simulink library "ros2lib"  (R2025a)
settings: Solver=ode45  StartTime=0.0  StopTime=10.0  RelTol=1e-3  EnableMultiTasking=on
undefined symbols (not defined in the file): coder, count, data, data_SL_Info, datatype, encoding, encoding_SL_Info, fields, fields_SL_Info, header, height, name, name_SL_Info, offset, point_step, ros, row_step, width
libraries: $bdroot x3
(part 2 of 2)

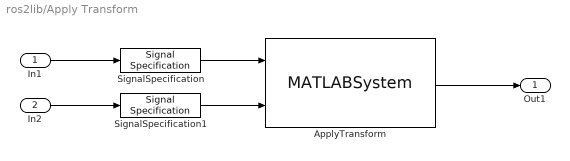
== system ros2lib/Apply Transform ==
  In1 : Inport
  In2 : Inport  Port=2
  ApplyTransform : MATLABSystem  System=ros.slros2.internal.block.ApplyTransform  EntityMsgType=geometry_msgs/QuaternionStamped  ModelName=ros2lib  BlockId=APTF_ros2lib_222  SLOutputBusName=SL_Bus_geometry_msgs_QuaternionStamped
      mask Type: ros.slros2.internal.block.ApplyTransform
  SignalSpecification : SignalSpecification  OutDataTypeStr=Bus: SL_Bus_geometry_msgs_TransformStamped  BusOutputAsStruct=on
      settings: LockScale=on
  SignalSpecification1 : SignalSpecification  OutDataTypeStr=Bus: SL_Bus_geometry_msgs_QuaternionStamped  BusOutputAsStruct=on
      settings: LockScale=on
  Out1 : Outport
  wires:
  In2/1 -> SignalSpecification1/1
  SignalSpecification1/1 -> ApplyTransform/2
  ApplyTransform/1 -> Out1/1
  In1/1 -> SignalSpecification/1
  SignalSpecification/1 -> ApplyTransform/1

== system ros2lib/Blank Message ==
  Constant : Constant  Value=0  OutDataTypeStr=Bus: SL_Bus_geometry_msgs_Point  SampleTime=SampleTime  LockScale=on
  Out : Outport  VectorParamsAs1DForOutWhenUnconnected=off  LockScale=on
  wires:
  Constant/1 -> Out/1

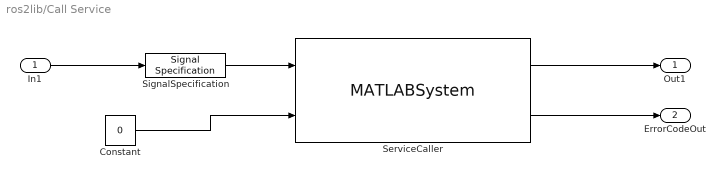
== system ros2lib/Call Service ==
  In1 : Inport
  Constant : Constant  Value=0  VectorParams1D=off  OutDataTypeStr=Bus: SL_Bus_std_srvs_EmptyResponse  SampleTime=-1
  ServiceCaller : MATLABSystem  System=ros.slros2.internal.block.ServiceCaller  QOSHistory=Keep last  QOSDepth=QOSDepth  QOSReliability=Reliable  QOSDurability=Volatile  QOSDeadline=QOSDeadline  QOSLifespan=QOSLifespan  QOSLiveliness=Automatic  QOSLeaseDuration=QOSLeaseDuration  ServiceName=/my_service  ServiceType=std_srvs/Empty  ConnectionTimeout=5  IsPersistentConnection=off  SLInputBusName=SL_Bus_std_srvs_EmptyRequest  SLOutputBusName=SL_Bus_std_srvs_EmptyResponse  ModelName=ros2lib  BlockId=ServCall_ros2lib_179
      mask Type: ros.slros2.internal.block.ServiceCaller
  SignalSpecification : SignalSpecification  OutDataTypeStr=Bus: SL_Bus_std_srvs_EmptyRequest  BusOutputAsStruct=on
      settings: LockScale=on
  Out1 : Outport
  ErrorCodeOut : Outport  Port=2
  wires:
  ServiceCaller/2 -> ErrorCodeOut/1
  Constant/1 -> ServiceCaller/2
  ServiceCaller/1 -> Out1/1
  In1/1 -> SignalSpecification/1
  SignalSpecification/1 -> ServiceCaller/1

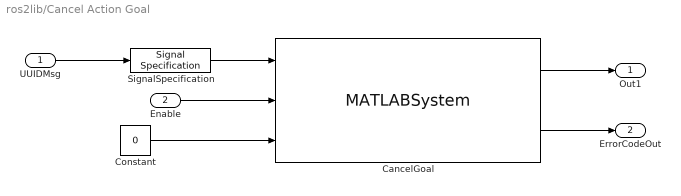
== system ros2lib/Cancel Action Goal ==
  UUIDMsg : Inport
  Enable : Inport  Port=2  OutDataTypeStr=boolean
  CancelGoal : MATLABSystem  System=ros.slros2.internal.block.CancelActionGoal  SLUUIDInputBusName=SL_Bus_unique_identifier_msgs_UUID  SLResponseOutputBusName=SL_Bus_action_msgs_CancelGoalResponse  ModelName=ros2lib  BlockId=ActCancel_ros2lib_244
      mask Type: ros.slros2.internal.block.CancelActionGoal
  Constant : Constant  Value=0  OutDataTypeStr=Bus: SL_Bus_action_msgs_CancelGoalResponse
  SignalSpecification : SignalSpecification  OutDataTypeStr=Bus: SL_Bus_unique_identifier_msgs_UUID  BusOutputAsStruct=on
      settings: LockScale=on
  Out1 : Outport
  ErrorCodeOut : Outport  Port=2
  wires:
  CancelGoal/2 -> ErrorCodeOut/1
  Constant/1 -> CancelGoal/3
  UUIDMsg/1 -> SignalSpecification/1
  Enable/1 -> CancelGoal/2
  SignalSpecification/1 -> CancelGoal/1
  CancelGoal/1 -> Out1/1

== system ros2lib/Get Transform ==
  Constant : Constant  Value=0  OutDataTypeStr=Bus: SL_Bus_geometry_msgs_TransformStamped  SampleTime=SampleTime
  SourceBlock : MATLABSystem  System=ros.slros2.internal.block.GetTransform  SLBusName=SL_Bus_geometry_msgs_TransformStamped  DynamicQoSHistory=Keep last  DynamicQoSDepth=DynamicQoSDepth  DynamicQoSReliability=Reliable  DynamicQoSDurability=Volatile  DynamicQOSDeadline=DynamicQoSDeadline  DynamicQOSLifespan=DynamicQoSLifespan  DynamicQOSLiveliness=Automatic  DynamicQOSLeaseDuration=DynamicQoSLeaseDuration  StaticQoSHistory=Keep last  StaticQoSDepth=StaticQoSDepth  StaticQoSReliability=Reliable  StaticQoSDurability=Volatile  StaticQOSDeadline=StaticQoSDeadline  StaticQOSLifespan=StaticQoSLifespan  StaticQOSLiveliness=Automatic  StaticQOSLeaseDuration=StaticQoSLeaseDuration  OutputFormat=bus  SampleTime=-1  ModelName=ros2lib  BlockId=TF_ros2lib_223
      mask Type: ros.slros2.internal.block.GetTransform
  Out1 : Outport
  Out2 : Outport  Port=2
  wires:
  Constant/1 -> SourceBlock/1
  SourceBlock/1 -> Out1/1
  SourceBlock/2 -> Out2/1

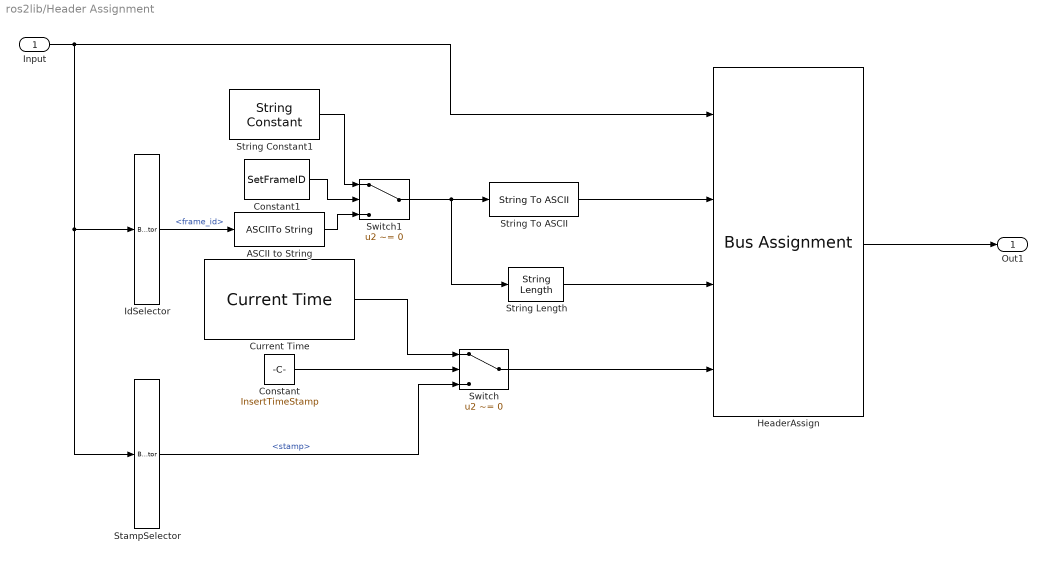
== system ros2lib/Header Assignment ==
  Input : Inport
  ASCII to String : ASCIIToString
  Constant : Constant  Value=InsertTimeStamp
  Constant1 : Constant  Value=SetFrameID
  Current Time : $bdroot/Current Time  OutputFormat=bus  SampleTime=-1  ModelName=tt
  HeaderAssign : BusAssignment  AssignedSignals=header.frame_id,header.frame_id_SL_Info.CurrentLength,header.stamp
  IdSelector : BusSelector  OutputSignals=header.frame_id
  StampSelector : BusSelector  OutputSignals=header.stamp
  String Constant1 : StringConstant  String=FrameID
  String Length : StringLength
  String To ASCII : StringToASCII  OutputVectorSize=128
  Switch : Switch  Criteria=u2 ~= 0  Threshold=1.5  SaturateOnIntegerOverflow=off  InputSameDT=off
  Switch1 : Switch  Criteria=u2 ~= 0  Threshold=1.5  SaturateOnIntegerOverflow=off  InputSameDT=off
  Out1 : Outport
  wires:
  Switch/1 -> HeaderAssign/4
  StampSelector/1 -> Switch/3  "<stamp>"
  Constant1/1 -> Switch1/2
  Constant/1 -> Switch/2
  String Length/1 -> HeaderAssign/3
  String Constant1/1 -> Switch1/1
  Switch1/1 -> String Length/1, String To ASCII/1
  Current Time/1 -> Switch/1
  String To ASCII/1 -> HeaderAssign/2
  ASCII to String/1 -> Switch1/3
  IdSelector/1 -> ASCII to String/1  "<frame_id>"
  HeaderAssign/1 -> Out1/1
  Input/1 -> StampSelector/1, IdSelector/1, HeaderAssign/1

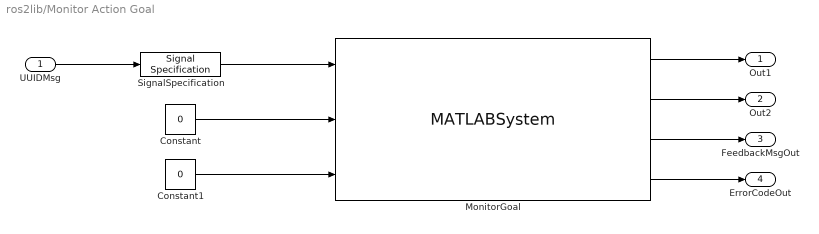
== system ros2lib/Monitor Action Goal ==
  UUIDMsg : Inport
  Constant : Constant  Value=0  OutDataTypeStr=Bus: SL_Bus_example_interfaces_FibonacciResult
  Constant1 : Constant  Value=0  OutDataTypeStr=Bus: SL_Bus_example_interfaces_FibonacciFeedback
  MonitorGoal : MATLABSystem  System=ros.slros2.internal.block.MonitorActionGoal  ActionName=/fibonacci  ActionType=example_interfaces/Fibonacci  SLUUIDInputBusName=SL_Bus_unique_identifier_msgs_UUID  SLFeedbackOutputBusName=SL_Bus_example_interfaces_FibonacciFeedback  SLResultOutputBusName=SL_Bus_example_interfaces_FibonacciResult  ModelName=ros2lib  BlockId=ActSend_ros2lib_226
      mask Type: ros.slros2.internal.block.MonitorActionGoal
  SignalSpecification : SignalSpecification  OutDataTypeStr=Bus: SL_Bus_unique_identifier_msgs_UUID  BusOutputAsStruct=on
      settings: LockScale=on
  Out1 : Outport
  Out2 : Outport  Port=2
  FeedbackMsgOut : Outport  Port=3
  ErrorCodeOut : Outport  Port=4
  wires:
  UUIDMsg/1 -> SignalSpecification/1
  Constant/1 -> MonitorGoal/2
  MonitorGoal/1 -> Out1/1
  MonitorGoal/2 -> Out2/1
  SignalSpecification/1 -> MonitorGoal/1
  MonitorGoal/3 -> FeedbackMsgOut/1
  Constant1/1 -> MonitorGoal/3
  MonitorGoal/4 -> ErrorCodeOut/1

== system ros2lib/Publish ==
  In1 : Inport  LockScale=on
  SignalSpecification : SignalSpecification  OutDataTypeStr=Bus: SL_Bus_geometry_msgs_Point  BusOutputAsStruct=on
      settings: LockScale=on
  SinkBlock : MATLABSystem  System=ros.slros2.internal.block.Publisher  QOSHistory=Keep last  QOSDepth=QOSDepth  QOSReliability=Reliable  QOSDurability=Volatile  QOSDeadline=QOSDeadline  QOSLifespan=QOSLifespan  QOSLiveliness=Automatic  QOSLeaseDuration=QOSLeaseDuration  ROSTopic=/my_topic  ROSMessageType=geometry_msgs/Point  SLBusName=SL_Bus_geometry_msgs_Point  ModelName=ros2lib  BlockId=Pub_ros2lib_156
      mask Type: ros.slros2.internal.block.Publisher
  wires:
  SignalSpecification/1 -> SinkBlock/1
  In1/1 -> SignalSpecification/1

== system ros2lib/Read Data ==
  SourceBlock : MATLABSystem  System=ros.slros2.internal.block.ReadData  LogfileType=rosbag2  Topic=/my_topic  SampleTime=sampleTime  ModelName=ros2lib
      mask Type: ros.slros2.internal.block.ReadData
  Out1 : Outport
  Out2 : Outport  Port=2
  wires:
  SourceBlock/2 -> Out2/1
  SourceBlock/1 -> Out1/1

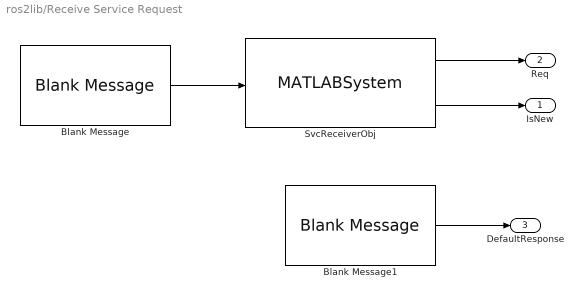
== system ros2lib/Receive Service Request ==
  Blank Message : $bdroot/Blank Message  messageClass=Service Request  entityType=std_srvs/Empty  messageType=std_srvs/EmptyRequest  SampleTime=SampleTime
  Blank Message1 : $bdroot/Blank Message  messageClass=Service Response  entityType=std_srvs/Empty  messageType=std_srvs/EmptyResponse  SampleTime=SampleTime
  SvcReceiverObj : MATLABSystem  System=ros.slros2.internal.block.SvcRequestReceiver  SLBusName=SL_Bus_std_srvs_EmptyRequest  ModelName=ros2lib  ServiceName=/my_service  ServiceType=std_srvs/Empty  BlockId=ServRec_ros2lib_224  QOSHistory=Keep last  QOSDepth=QOSDepth  QOSReliability=Reliable  QOSDurability=Volatile  QOSDeadline=QOSDeadline  QOSLifespan=QOSLifespan  QOSLiveliness=Automatic  QOSLeaseDuration=QOSLeaseDuration
      mask Type: ros.slros2.internal.block.SvcRequestReceiver
  IsNew : Outport
  Req : Outport  Port=2
  DefaultResponse : Outport  Port=3
  wires:
  Blank Message1/1 -> DefaultResponse/1
  Blank Message/1 -> SvcReceiverObj/1
  SvcReceiverObj/1 -> Req/1
  SvcReceiverObj/2 -> IsNew/1

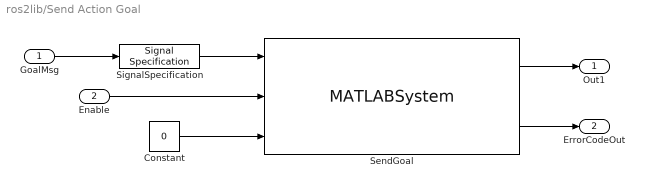
== system ros2lib/Send Action Goal ==
  GoalMsg : Inport
  Enable : Inport  Port=2  OutDataTypeStr=boolean
  Constant : Constant  Value=0  OutDataTypeStr=Bus: SL_Bus_unique_identifier_msgs_UUID
  SendGoal : MATLABSystem  System=ros.slros2.internal.block.SendActionGoal  ActionType=example_interfaces/Fibonacci  OutputROSMessageType=unique_identifier_msgs/UUID  SLUUIDOutputBusName=SL_Bus_unique_identifier_msgs_UUID  GoalServiceQoSHistory=Keep last  GoalServiceQoSDepth=GoalServiceQoSDepth  GoalServiceQoSReliability=Reliable  GoalServiceQoSDurability=Volatile  GoalServiceQoSDeadline=GoalServiceQoSDeadline  GoalServiceQoSLifespan=GoalServiceQoSLifespan  GoalServiceQoSLiveliness=Automatic  GoalServiceQoSLeaseDuration=GoalServiceQoSLeaseDuration  ResultServiceQoSHistory=Keep last  ResultServiceQoSDepth=ResultServiceQoSDepth  ResultServiceQoSReliability=Reliable  ResultServiceQoSDurability=Volatile  ResultServiceQoSDeadline=ResultServiceQoSDeadline  ResultServiceQoSLifespan=ResultServiceQoSLifespan  ResultServiceQoSLiveliness=Automatic  ResultServiceQoSLeaseDuration=ResultServiceQoSLeaseDuration  CancelServiceQoSHistory=Keep last  CancelServiceQoSDepth=CancelServiceQoSDepth  CancelServiceQoSReliability=Reliable  CancelServiceQoSDurability=Volatile  CancelServiceQoSDeadline=CancelServiceQoSDeadline  CancelServiceQoSLifespan=CancelServiceQoSLifespan  CancelServiceQoSLiveliness=Automatic  CancelServiceQoSLeaseDuration=CancelServiceQoSLeaseDuration  FeedbackTopicQoSHistory=Keep last  FeedbackTopicQoSDepth=FeedbackTopicQoSDepth  FeedbackTopicQoSReliability=Reliable  FeedbackTopicQoSDurability=Volatile  FeedbackTopicQoSDeadline=FeedbackTopicQoSDeadline  FeedbackTopicQoSLifespan=FeedbackTopicQoSLifespan  FeedbackTopicQoSLiveliness=Automatic  FeedbackTopicQoSLeaseDuration=FeedbackTopicQoSLeaseDuration  StatusTopicQoSHistory=Keep last  StatusTopicQoSDepth=StatusTopicQoSDepth  StatusTopicQoSReliability=Reliable  StatusTopicQoSDurability=Transient local  StatusTopicQoSDeadline=StatusTopicQoSDeadline  StatusTopicQoSLifespan=StatusTopicQoSLifespan  StatusTopicQoSLiveliness=Automatic  StatusTopicQoSLeaseDuration=StatusTopicQoSLeaseDuration  ActionName=/fibonacci  SLGoalInputBusName=SL_Bus_example_interfaces_FibonacciGoal  ModelName=ros2lib  BlockId=ActSend_ros2lib_226
      mask Type: ros.slros2.internal.block.SendActionGoal
  SignalSpecification : SignalSpecification  OutDataTypeStr=Bus: SL_Bus_example_interfaces_FibonacciGoal  BusOutputAsStruct=on
      settings: LockScale=on
  Out1 : Outport
  ErrorCodeOut : Outport  Port=2
  wires:
  SendGoal/1 -> Out1/1
  Constant/1 -> SendGoal/3
  SignalSpecification/1 -> SendGoal/1
  Enable/1 -> SendGoal/2
  GoalMsg/1 -> SignalSpecification/1
  SendGoal/2 -> ErrorCodeOut/1

== system ros2lib/Send Service Response ==
  resp : Inport
  SignalSpecification : SignalSpecification  OutDataTypeStr=Bus: SL_Bus_std_srvs_EmptyResponse  BusOutputAsStruct=on
      settings: LockScale=on
  SvcSenderObj : MATLABSystem  System=ros.slros2.internal.block.SvcResponseSender  ModelName=ros2lib  ServiceName=/my_service  ServiceType=std_srvs/Empty  BlockId=ServRec_ros2lib_224
      mask Type: ros.slros2.internal.block.SvcResponseSender
  wires:
  SignalSpecification/1 -> SvcSenderObj/1
  resp/1 -> SignalSpecification/1

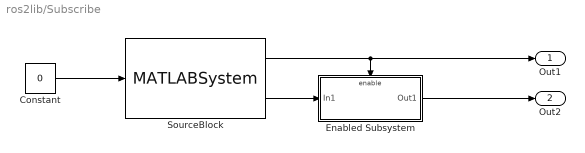
== system ros2lib/Subscribe ==
  Constant : Constant  Value=0  OutDataTypeStr=Bus: SL_Bus_geometry_msgs_Point  SampleTime=sampleTime  LockScale=on
  Enabled Subsystem : Subsystem  TreatAsAtomicUnit=on
  SourceBlock : MATLABSystem  System=ros.slros2.internal.block.Subscriber  QOSHistory=Keep last  QOSDepth=QOSDepth  QOSReliability=Reliable  QOSDurability=Volatile  QOSDeadline=QOSDeadline  QOSLifespan=QOSLifespan  QOSLiveliness=Automatic  QOSLeaseDuration=QOSLeaseDuration  ROSTopic=/my_topic  ROSMessageType=geometry_msgs/Point  SLBusName=SL_Bus_geometry_msgs_Point  ModelName=ros2lib  BlockId=Sub_ros2lib_139
      mask Type: ros.slros2.internal.block.Subscriber
  Out1 : Outport  VectorParamsAs1DForOutWhenUnconnected=off
  Out2 : Outport  Port=2  VectorParamsAs1DForOutWhenUnconnected=off
  wires:
  SourceBlock/1 -> Enabled Subsystem/Enable, Out1/1
  SourceBlock/2 -> Enabled Subsystem/1(In1)
  Constant/1 -> SourceBlock/1
  Enabled Subsystem/1(Out1) -> Out2/1

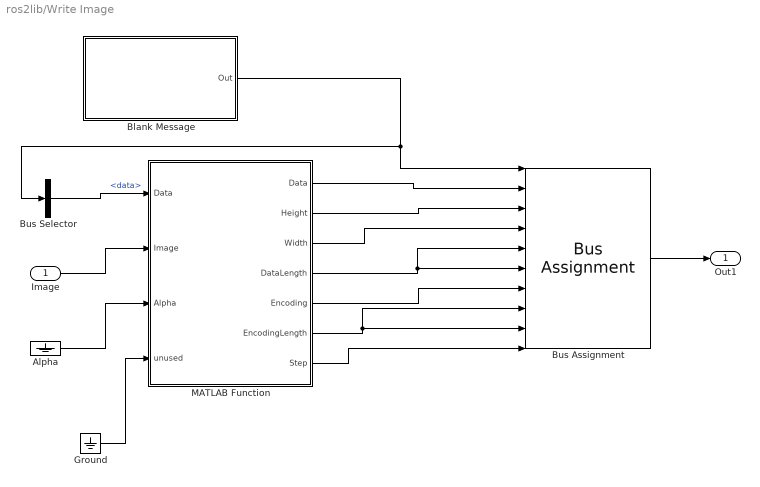
== system ros2lib/Write Image ==
  Image : Inport
  Alpha : Ground
  Blank Message : Subsystem  LoadFcn=ros.slros2.internal.block.MessageBlockMask.messageLoadFcn(gcb);  InitFcn=ros.slros.internal.block.errorIfBlocksConflict(bdroot(gcb));  mask(ROS2 Blank Message){messageClass=Message, entityType=sensor_msgs/Image, messageType=sensor_msgs/Image, SampleTime=inf}
      mask prompts: messageClass "ros:slros:blockmask:MessageClassPrompt"; entityType "ros:slros:blockmask:TypePrompt"; messageType "ros:slros:blockmask:FullTypePrompt"; SampleTime "Simulink:blkprm_prompts:AllSrcBlksSampleTime"
      mask help: ros:slros2:blockmask:BlankMsgDescription
      mask init:
      | ros.slros2.internal.block.MessageBlockMask.dispatch('maskInitialize', gcb);
      settings: ModelCloseFcn=ros.slros2.internal.bus.Util.clearSLBusesInGlobalScope();
      mask Help: eval('ros.slros.internal.helpview(''ros2BlankMsgBlock'')');
      mask TypeOptions messageClass: ros:slros:blockmask:MessageType_Msg | ros:slros:blockmask:MessageType_SrvReq | ros:slros:blockmask:MessageType_SrvResp
      mask Callback messageClass: ros.slros2.internal.block.MessageBlockMask.dispatch('messageClassChange', gcb);
      mask Callback entityType: ros.slros2.internal.block.MessageBlockMask.dispatch('entityTypeEdit', gcb);
      mask TypeOptions SampleTime: Constant/SampleTime
      mask DialogControl messageClass Prompt: Class:
      mask DialogControl entityType Prompt: Type:
      mask DialogControl id_msgTypeSelectBtn Prompt: ros:slros:blockmask:SelectPrompt
      mask DialogControl id_msgTypeSelectBtn Callback: ros.slros2.internal.block.MessageBlockMask.dispatch('selectButtonPressed', gcb);
      mask DialogControl messageType Prompt: Fully resolved type:
      mask DialogControl SampleTime Prompt: Sample time:
      mask Display: color('black');
  Bus Assignment : BusAssignment  AssignedSignals=data,height,width,data_SL_Info.CurrentLength,data_SL_Info.ReceivedLength,encoding,encoding_SL_Info.CurrentLength,encoding_SL_Info.ReceivedLength,step
  Bus Selector : BusSelector  OutputSignals=data
  Ground : Ground
  MATLAB Function : MATLAB Function  TreatAsAtomicUnit=on
  Out1 : Outport
  wires:
  MATLAB Function/1(Data) -> Bus Assignment/2
  MATLAB Function/3(Width) -> Bus Assignment/4
  MATLAB Function/5(Encoding) -> Bus Assignment/7
  Blank Message/1(Out) -> Bus Selector/1, Bus Assignment/1
  Bus Assignment/1 -> Out1/1
  MATLAB Function/2(Height) -> Bus Assignment/3
  Bus Selector/1 -> MATLAB Function/1("Data ")  "<data>"
  MATLAB Function/7(Step) -> Bus Assignment/10
  MATLAB Function/6(EncodingLength) -> Bus Assignment/8, Bus Assignment/9
  MATLAB Function/4(DataLength) -> Bus Assignment/5, Bus Assignment/6
  Image/1 -> MATLAB Function/2(Image)
  Alpha/1 -> MATLAB Function/3(Alpha)
  Ground/1 -> MATLAB Function/4(unused)

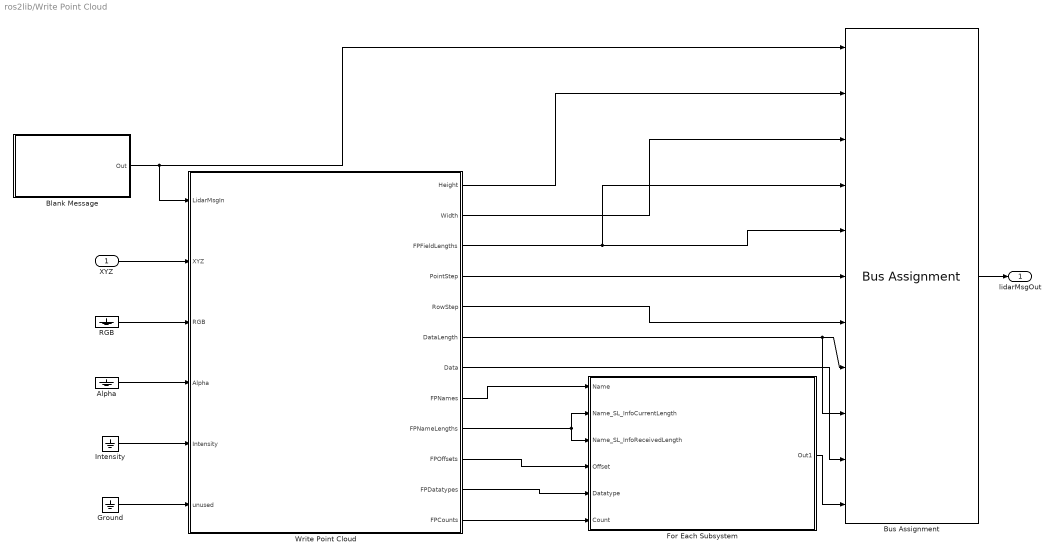
== system ros2lib/Write Point Cloud ==
  XYZ : Inport
  Alpha : Ground
  Blank Message : Subsystem  LoadFcn=ros.slros2.internal.block.MessageBlockMask.messageLoadFcn(gcb);  InitFcn=ros.slros.internal.block.errorIfBlocksConflict(bdroot(gcb));  mask(ROS2 Blank Message){messageClass=Message, entityType=sensor_msgs/PointCloud2, messageType=sensor_msgs/PointCloud2, SampleTime=inf}
      mask prompts: messageClass "ros:slros:blockmask:MessageClassPrompt"; entityType "ros:slros:blockmask:TypePrompt"; messageType "ros:slros:blockmask:FullTypePrompt"; SampleTime "Simulink:blkprm_prompts:AllSrcBlksSampleTime"
      mask help: ros:slros2:blockmask:BlankMsgDescription
      mask init:
      | ros.slros2.internal.block.MessageBlockMask.dispatch('maskInitialize', gcb);
      settings: ModelCloseFcn=ros.slros2.internal.bus.Util.clearSLBusesInGlobalScope();
      mask Help: eval('ros.slros.internal.helpview(''ros2BlankMsgBlock'')');
      mask TypeOptions messageClass: ros:slros:blockmask:MessageType_Msg | ros:slros:blockmask:MessageType_SrvReq | ros:slros:blockmask:MessageType_SrvResp
      mask Callback messageClass: ros.slros2.internal.block.MessageBlockMask.dispatch('messageClassChange', gcb);
      mask Callback entityType: ros.slros2.internal.block.MessageBlockMask.dispatch('entityTypeEdit', gcb);
      mask TypeOptions SampleTime: Constant/SampleTime
      mask DialogControl messageClass Prompt: Class:
      mask DialogControl entityType Prompt: Type:
      mask DialogControl id_msgTypeSelectBtn Prompt: ros:slros:blockmask:SelectPrompt
      mask DialogControl id_msgTypeSelectBtn Callback: ros.slros2.internal.block.MessageBlockMask.dispatch('selectButtonPressed', gcb);
      mask DialogControl messageType Prompt: Fully resolved type:
      mask DialogControl SampleTime Prompt: Sample time:
      mask Display: color('black');
  Bus Assignment : BusAssignment  AssignedSignals=height,width,fields_SL_Info.CurrentLength,fields_SL_Info.ReceivedLength,point_step,row_step,data_SL_Info.CurrentLength,data_SL_Info.ReceivedLength,data,fields
  For Each Subsystem : Subsystem  TreatAsAtomicUnit=on
  Ground : Ground
  Intensity : Ground
  RGB : Ground
  Write Point Cloud : MATLAB Function  TreatAsAtomicUnit=on
  lidarMsgOut : Outport
  wires:
  Bus Assignment/1 -> lidarMsgOut/1
  Write Point Cloud/12(FPCounts) -> For Each Subsystem/6(Count)
  Write Point Cloud/11(FPDatatypes) -> For Each Subsystem/5(Datatype)
  Write Point Cloud/10(FPOffsets) -> For Each Subsystem/4(Offset)
  Write Point Cloud/9(FPNameLengths) -> For Each Subsystem/2(Name_SL_InfoCurrentLength), For Each Subsystem/3(Name_SL_InfoReceivedLength)
  Write Point Cloud/8(FPNames) -> For Each Subsystem/1(Name)
  Write Point Cloud/7(Data) -> Bus Assignment/10
  For Each Subsystem/1(Out1) -> Bus Assignment/11
  Write Point Cloud/6(DataLength) -> Bus Assignment/8, Bus Assignment/9
  Write Point Cloud/5(RowStep) -> Bus Assignment/7
  Write Point Cloud/3(FPFieldLengths) -> Bus Assignment/5, Bus Assignment/4
  Intensity/1 -> Write Point Cloud/5(Intensity)
  Alpha/1 -> Write Point Cloud/4(Alpha)
  Ground/1 -> Write Point Cloud/6(unused)
  Write Point Cloud/2(Width) -> Bus Assignment/3
  RGB/1 -> Write Point Cloud/3(RGB)
  Write Point Cloud/1(Height) -> Bus Assignment/2
  Blank Message/1(Out) -> Write Point Cloud/1(LidarMsgIn), Bus Assignment/1
  XYZ/1 -> Write Point Cloud/2(XYZ)
  Write Point Cloud/4(PointStep) -> Bus Assignment/6

== system ros2lib/Subscribe/Enabled Subsystem ==
  note: In Enable block, States when enabling = "held".
      | This ensures the "latch" behavior, i.e., this subsystem
      | will output its input when enabled, and its most recent
      | valid input when disabled.
  note: In Outport bloc, Initial output on outport is 0.
      | This ensures that bus is zeroed out
      | (as the initial condition)
  In1 : Inport
  Enable : EnablePort
  Out1 : Outport  InitialOutput=0  VectorParamsAs1DForOutWhenUnconnected=off
  wires:
  In1/1 -> Out1/1

== system ros2lib/Write Image/Blank Message ==
  Constant : Constant  Value=0  OutDataTypeStr=Bus: SL_Bus_sensor_msgs_Image  SampleTime=SampleTime  LockScale=on
  Out : Outport  VectorParamsAs1DForOutWhenUnconnected=off  LockScale=on
  wires:
  Constant/1 -> Out/1

== system ros2lib/Write Point Cloud/Blank Message ==
  Constant : Constant  Value=0  OutDataTypeStr=Bus: SL_Bus_sensor_msgs_PointCloud2  SampleTime=SampleTime  LockScale=on
  Out : Outport  VectorParamsAs1DForOutWhenUnconnected=off  LockScale=on
  wires:
  Constant/1 -> Out/1

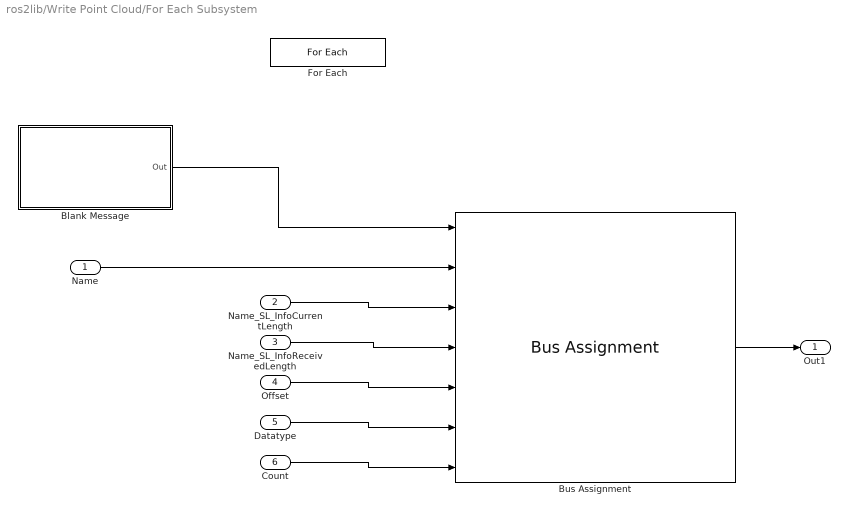
== system ros2lib/Write Point Cloud/For Each Subsystem ==
  Name : Inport  Partition=on  PartitionDimension=1  PartitionWidth=ros.slros.internal.bus.Util.getCurrentFieldLength('sensor_msgs/PointField','name','ros2')  PartitionOffset=0
  Name_SL_InfoCurrentLength : Inport  Port=2  Partition=on  PartitionDimension=1  PartitionWidth=1  PartitionOffset=0
  Name_SL_InfoReceivedLength : Inport  Port=3  Partition=on  PartitionDimension=1  PartitionWidth=1  PartitionOffset=0
  Offset : Inport  Port=4  Partition=on  PartitionDimension=1  PartitionWidth=1  PartitionOffset=0
  Datatype : Inport  Port=5  Partition=on  PartitionDimension=1  PartitionWidth=1  PartitionOffset=0
  Count : Inport  Port=6  Partition=on  PartitionDimension=1  PartitionWidth=1  PartitionOffset=0
  Blank Message : Subsystem  LoadFcn=ros.slros2.internal.block.MessageBlockMask.messageLoadFcn(gcb);  InitFcn=ros.slros.internal.block.errorIfBlocksConflict(bdroot(gcb));  mask(ROS2 Blank Message){messageClass=Message, entityType=sensor_msgs/PointField, messageType=sensor_msgs/PointField, SampleTime=inf}
      mask prompts: messageClass "ros:slros:blockmask:MessageClassPrompt"; entityType "ros:slros:blockmask:TypePrompt"; messageType "ros:slros:blockmask:FullTypePrompt"; SampleTime "Simulink:blkprm_prompts:AllSrcBlksSampleTime"
      mask help: ros:slros2:blockmask:BlankMsgDescription
      mask init:
      | ros.slros2.internal.block.MessageBlockMask.dispatch('maskInitialize', gcb);
      settings: ModelCloseFcn=ros.slros2.internal.bus.Util.clearSLBusesInGlobalScope();
      mask Help: eval('ros.slros.internal.helpview(''ros2BlankMsgBlock'')');
      mask TypeOptions messageClass: ros:slros:blockmask:MessageType_Msg | ros:slros:blockmask:MessageType_SrvReq | ros:slros:blockmask:MessageType_SrvResp
      mask Callback messageClass: ros.slros2.internal.block.MessageBlockMask.dispatch('messageClassChange', gcb);
      mask Callback entityType: ros.slros2.internal.block.MessageBlockMask.dispatch('entityTypeEdit', gcb);
      mask TypeOptions SampleTime: Constant/SampleTime
      mask DialogControl messageClass Prompt: Class:
      mask DialogControl entityType Prompt: Type:
      mask DialogControl id_msgTypeSelectBtn Prompt: ros:slros:blockmask:SelectPrompt
      mask DialogControl id_msgTypeSelectBtn Callback: ros.slros2.internal.block.MessageBlockMask.dispatch('selectButtonPressed', gcb);
      mask DialogControl messageType Prompt: Fully resolved type:
      mask DialogControl SampleTime Prompt: Sample time:
      mask Display: color('black');
  Bus Assignment : BusAssignment  AssignedSignals=name,name_SL_Info.CurrentLength,name_SL_Info.ReceivedLength,offset,datatype,count
  For Each : ForEach  DisableCoverage=on
  Out1 : Outport  ConcatenationDimension=1
  wires:
  Name/1 -> Bus Assignment/2
  Count/1 -> Bus Assignment/7
  Datatype/1 -> Bus Assignment/6
  Offset/1 -> Bus Assignment/5
  Name_SL_InfoReceivedLength/1 -> Bus Assignment/4
  Name_SL_InfoCurrentLength/1 -> Bus Assignment/3
  Bus Assignment/1 -> Out1/1
  Blank Message/1(Out) -> Bus Assignment/1

== system ros2lib/Write Point Cloud/For Each Subsystem/Blank Message ==
  Constant : Constant  Value=0  OutDataTypeStr=Bus: SL_Bus_sensor_msgs_PointField  SampleTime=SampleTime  LockScale=on
  Out : Outport  VectorParamsAs1DForOutWhenUnconnected=off  LockScale=on
  wires:
  Constant/1 -> Out/1

== matlab function ros2lib/Write Point Cloud/Write Point Cloud ==
  data: LidarMsgIn input; XYZ input; RGB input; Alpha input; Intensity input; unused input; FieldNamesStruct parameter; HasRGB parameter; HasAlpha parameter; Height output; Width output; FPFieldLengths output; PointStep output; RowStep output; DataLength output; Data output; FPNames output; FPNameLengths output; FPOffsets output; FPDatatypes output; FPCounts output; HasIntensity parameter
function [Height, Width, FPFieldLengths, PointStep, ...
    RowStep, DataLength, Data, FPNames,...
    FPNameLengths, FPOffsets, FPDatatypes, FPCounts] ...
    = WritePointCloudFcnBlock(LidarMsgIn, XYZ, RGB, Alpha, Intensity, ~, FieldNamesStruct, HasRGB, HasAlpha, HasIntensity)

unstructured = ismatrix(XYZ); 

MaxDataLength = length(LidarMsgIn.data);
NumFields = length(LidarMsgIn.fields);
NameLength = length(LidarMsgIn.fields(1).name);

[Height, Width, FPFieldLengths, PointStep, RowStep, DataLength, Data,   ...
    FPNames, FPNameLengths, FPOffsets, FPDatatypes, FPCounts] =         ...
    ros.internal.block.WritePointCloudFcnBlock(MaxDataLength, NumFields,...
    NameLength, XYZ, RGB, Alpha, Intensity, unstructured, HasRGB,       ...
    HasAlpha, HasIntensity, FieldNamesStruct, 'ROS2');

== matlab function ros2lib/Write Image/MATLAB Function ==
  data: Data input; Image input; Alpha input; unused input; Data output; Height output; Width output; DataLength output; Encoding output; EncodingLength output; Step output; EncodingStruct parameter; ImageEncoding parameter; HasAlpha parameter
function [Data, Height, Width, DataLength, Encoding, EncodingLength, Step]...
    = WriteImageFcnBlock(Data, Image, Alpha, ~, EncodingStruct, ImageEncoding, HasAlpha)
SelectedEncodingInd = ImageEncoding;
% Image encoding is set to evaluate in the mask,
% so the value is an index.
SelectedEncoding = ros.msg.sensor_msgs.internal.ImageEncoding.AllEncodings{SelectedEncodingInd};
type = EncodingStruct.DataType;
alphaSize = int32(size(Alpha));
imageSize = int32(size(Image));
% check types
if HasAlpha && ~isa(Alpha, type)
coder.internal.error('ros:slros2:image:InvalidAlphaType', SelectedEncoding, type)
elseif HasAlpha && ~ismatrix(Alpha)
coder.internal.error('ros:slros2:image:InvalidAlphaSize')
elseif ~isa(Image, type)
coder.internal.error('ros:slros2:image:InvalidImageType', SelectedEncoding, type)
end
if HasAlpha
    % check sizes
    if ~(imageSize(1) == alphaSize(1) && imageSize(2) == alphaSize(2))
        coder.internal.error('ros:slros2:image:IncompatibleImageAlphaSizes', ...
        fprintf("[%i, %i, %i]", imageSize(1), imageSize(2), imageSize(3)), ...
        fprintf("[%i, %i]", alphaSize(1), alphaSize(2)) )
    end

    ImageInput = cat(3, Image, Alpha);
else
    ImageInput = Image;
end
[Data, Height, Width, DataLength, Encoding, EncodingLength, Step]...
    = ros.internal.block.WriteImageFcnBlock(ImageInput, Data, EncodingStruct, SelectedEncodingInd);
